simulink model "HW_3sim"  (R2015a)
settings: Solver=ode45  StartTime=0.0  StopTime=tf  RelTol=1e-3
values from neighbouring files (symbols this model uses):
  F = [0,0,0,1,0,0;0,0,0,0,1,0;0,0,0,0,0,1; 3*n^2, 0, 0,0,2*n,0;0,0,0,-2*n,0,0;0,0,-n*n,0,0,0]    [hw_3.m]
  G = [0,0,0;0,0,0;0,0,0;1,0,0;0,1,0;0,0,1]    [hw_3.m]
  X0 = Xt(:,ind)'    [hw_3.m]
settings Model: Creator=avivpr  LastModifiedBy=avivpr

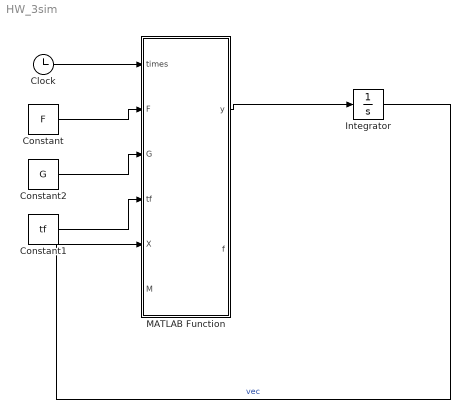
== system HW_3sim ==
  Clock : Clock
  Constant : Constant  Value=F
  Constant1 : Constant  Value=tf
  Constant2 : Constant  Value=G
  Integrator : Integrator  InitialCondition=X0
  MATLAB Function : MATLAB Function  TreatAsAtomicUnit=on
  wires:
  MATLAB Function/1(y) -> Integrator/1
  Integrator/1 -> MATLAB Function/5(X)  "vec"
  Clock/1 -> MATLAB Function/1(times)
  Constant/1 -> MATLAB Function/2(F)
  Constant2/1 -> MATLAB Function/3(G)
  Constant1/1 -> MATLAB Function/4(tf)

== matlab function HW_3sim/MATLAB Function ==
  data: times input; y output; F input; G input; tf input; X input; f output; M input
function [y,f]= fcn(times,F,G,tf,X,M)
f=zeros(2,1);
X_dot=zeros(4,1);
Mf=double(subs(M,t,tf-times));
K=G2'*expm(F'*(tf-times))*(inv(Mf*expm(F'*(tf-times)))*expm(F*(tf-times)));
f=K*X;
X_dot=(G*K+F)*X;







y = u;
